simulink model "A8_Problem_1"  (R2023b)
settings: Solver=VariableStepAuto  StartTime=0.0  StopTime=t  FixedStep=dt  RelTol=1e-3
undefined symbols (not defined in the file): A1, A2, alpha, angle_threshold, beta, g, Gamma, K, k, l, lambda_0, lambda_1, m, q_0, q_dot_0, sat_limit, switch_time, theta_0, useEstimates, w1, w2
settings Model: Creator=eliasoa  LastModifiedBy=eliasoa

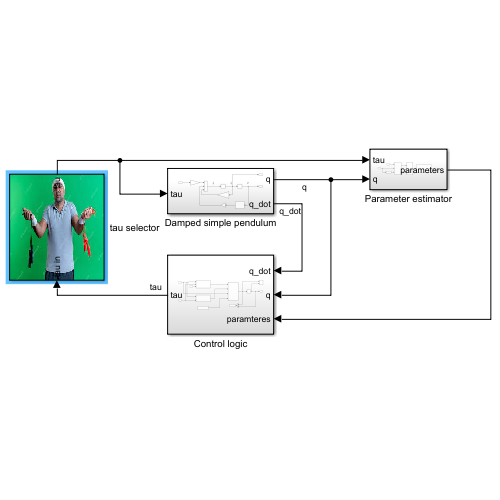
[thumbnail: Simulink's stored preview of the top-level diagram]
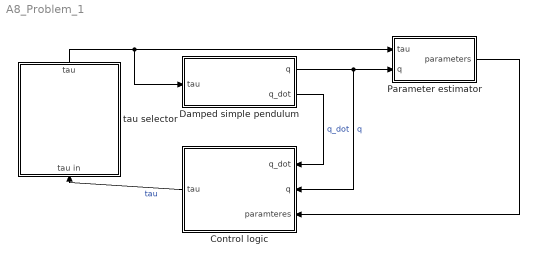
== system A8_Problem_1 ==
  Control logic : Subsystem
  Damped simple pendulum : Subsystem
  Parameter estimator : Subsystem
  "tau selector " : Subsystem
      mask Display: image('two tau.jpg');
  wires:
  Damped simple pendulum/1(q) -> Control logic/2(q), Parameter estimator/2(q)  "q"
  Damped simple pendulum/2(q_dot) -> Control logic/1(q_dot)  "q_dot"
  Parameter estimator/1(parameters) -> Control logic/3(paramteres)
  "tau selector "/1(tau) -> Damped simple pendulum/1(tau), Parameter estimator/1(tau)
  Control logic/1(tau) -> "tau selector "/1(tau in)  "tau"

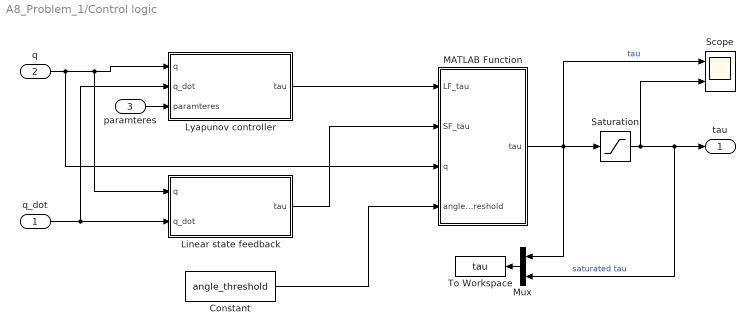
== system A8_Problem_1/Control logic ==
  q_dot : Inport
  q : Inport  Port=2
  paramteres : Inport  Port=3
  Constant : Constant  Value=angle_threshold
  Linear state feedback : Subsystem
  Lyapunov controller : Subsystem
  MATLAB Function : MATLAB Function  TreatAsAtomicUnit=on
  Mux : Mux  Inputs=2
  Saturation : Saturate  UpperLimit=sat_limit  LowerLimit=-sat_limit
  Scope : Scope  NumInputPorts=2
  To Workspace : ToWorkspace  VariableName=tau  SaveFormat=Timeseries  SampleTime=-1
  tau : Outport
  wires:
  q/1 -> Lyapunov controller/1(q), Linear state feedback/1(q), MATLAB Function/3(q)
  q_dot/1 -> Lyapunov controller/2(q_dot), Linear state feedback/2(q_dot)
  Linear state feedback/1(tau) -> MATLAB Function/2(SF_tau)
  Lyapunov controller/1(tau) -> MATLAB Function/1(LF_tau)
  MATLAB Function/1(tau) -> Saturation/1, Mux/1, Scope/1  "tau"
  Saturation/1 -> Scope/2, Mux/2, tau/1  "saturated tau"
  Mux/1 -> To Workspace/1
  Constant/1 -> MATLAB Function/4(angle_threshold)
  paramteres/1 -> Lyapunov controller/3(paramteres)

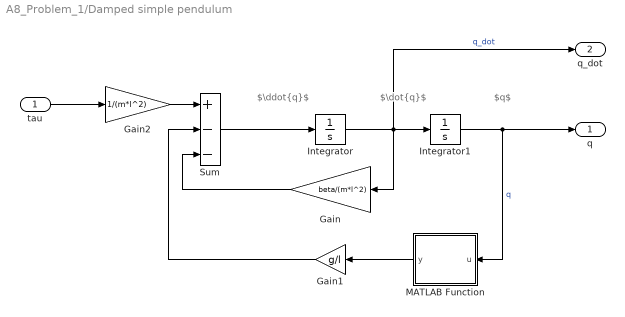
== system A8_Problem_1/Damped simple pendulum ==
  note: $\ddot{q}$
  note: $\dot{q}$
  note: $q$
  tau : Inport
  Gain : Gain  Gain=beta/(m*l^2)
  Gain1 : Gain  Gain=g/l
  Gain2 : Gain  Gain=1/(m*l^2)
  Integrator : Integrator  InitialCondition=q_dot_0
  Integrator1 : Integrator  InitialCondition=q_0
  MATLAB Function : MATLAB Function  TreatAsAtomicUnit=on
  Sum : Sum  Inputs=+--
  q : Outport
  q_dot : Outport  Port=2
  wires:
  tau/1 -> Gain2/1
  Sum/1 -> Integrator/1
  Gain2/1 -> Sum/1
  Gain/1 -> Sum/3
  MATLAB Function/1(y) -> Gain1/1
  Gain1/1 -> Sum/2
  Integrator/1 -> Integrator1/1, q_dot/1, Gain/1  "q_dot"
  Integrator1/1 -> q/1, MATLAB Function/1(u)  "q"

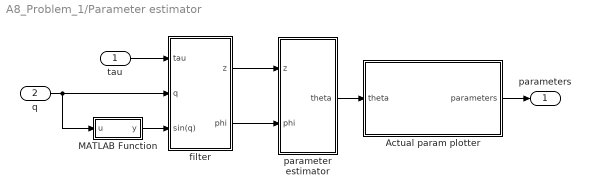
== system A8_Problem_1/Parameter estimator ==
  tau : Inport
  q : Inport  Port=2
  Actual param plotter : Subsystem
      mask Display: image('Kowalski.jpg');
  MATLAB Function : MATLAB Function  TreatAsAtomicUnit=on
  filter : Subsystem
  parameter estimator : Subsystem
  parameters : Outport
  wires:
  q/1 -> MATLAB Function/1(u), filter/2(q)
  tau/1 -> filter/1(tau)
  parameter estimator/1(theta) -> Actual param plotter/1(theta)
  filter/2(phi) -> parameter estimator/2(phi)
  Actual param plotter/1(parameters) -> parameters/1
  filter/1(z) -> parameter estimator/1(z)
  MATLAB Function/1(y) -> filter/3(sin(q))

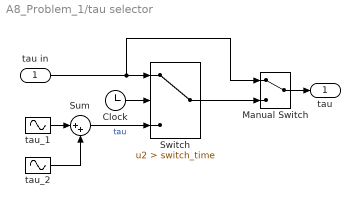
== system A8_Problem_1/tau selector  ==
  tau in : Inport
  Clock : Clock
  Manual Switch : ManualSwitch
  Sum : Sum  Inputs=|++
  Switch : Switch  Criteria=u2 > Threshold  Threshold=switch_time  SaturateOnIntegerOverflow=off  InputSameDT=off
  tau_1 : Sin  Amplitude=A1  Frequency=w1  SampleTime=0
  tau_2 : Sin  Amplitude=A2  Frequency=w2  SampleTime=0
  tau : Outport
  wires:
  tau in/1 -> Manual Switch/1, Switch/1
  tau_2/1 -> Sum/2
  tau_1/1 -> Sum/1
  Switch/1 -> Manual Switch/2
  Sum/1 -> Switch/3  "tau"
  Clock/1 -> Switch/2
  Manual Switch/1 -> tau/1

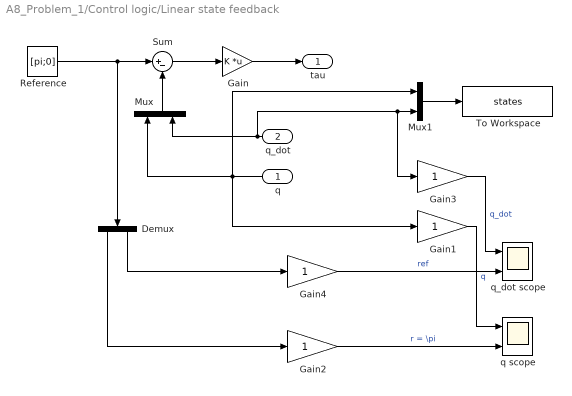
== system A8_Problem_1/Control logic/Linear state feedback ==
  q : Inport
  q_dot : Inport  Port=2
  Demux : Demux  Outputs=2
  Gain : Gain  Gain=K  Multiplication=Matrix(K*u)
  Gain{1..4} (4 alike) : Gain
  Mux : Mux  Inputs=2
  Mux1 : Mux  Inputs=2
  Reference : Constant  Value=[pi;0]
  Sum : Sum  Inputs=|+-
  To Workspace : ToWorkspace  VariableName=states  SaveFormat=Timeseries  SampleTime=-1
  q scope : Scope  NumInputPorts=2
  q_dot scope : Scope  NumInputPorts=2
  tau : Outport
  wires:
  Sum/1 -> Gain/1
  Mux/1 -> Sum/2
  Demux/2 -> Gain4/1
  q_dot/1 -> Gain3/1, Mux1/2, Mux/2
  q/1 -> Gain1/1, Mux/1, Mux1/1
  Demux/1 -> Gain2/1
  Reference/1 -> Sum/1, Demux/1
  Gain1/1 -> q scope/1  "q"
  Gain2/1 -> q scope/2  "r = \\pi"
  Gain/1 -> tau/1
  Mux1/1 -> To Workspace/1
  Gain4/1 -> q_dot scope/2  "ref"
  Gain3/1 -> q_dot scope/1  "q_dot"

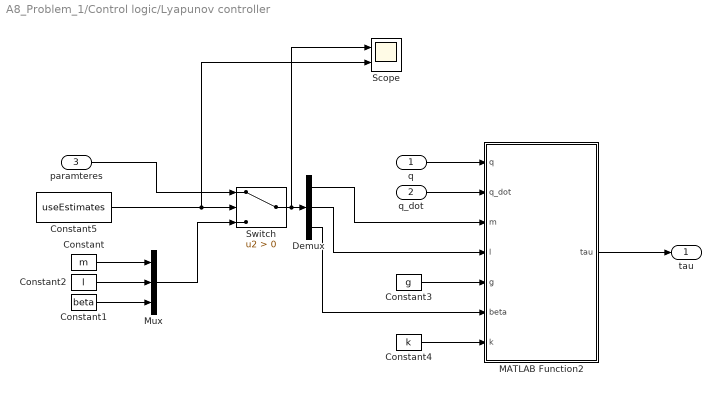
== system A8_Problem_1/Control logic/Lyapunov controller ==
  q : Inport
  q_dot : Inport  Port=2
  paramteres : Inport  Port=3
  Constant : Constant  Value=m
  Constant1 : Constant  Value=beta
  Constant2 : Constant  Value=l
  Constant3 : Constant  Value=g
  Constant4 : Constant  Value=k
  Constant5 : Constant  Value=useEstimates
  Demux : Demux  Outputs=3
  MATLAB Function2 : MATLAB Function  TreatAsAtomicUnit=on
  Mux : Mux  Inputs=3
  Scope : Scope  NumInputPorts=2
  Switch : Switch  Criteria=u2 > Threshold  SaturateOnIntegerOverflow=off  InputSameDT=off
  tau : Outport
  wires:
  MATLAB Function2/1(tau) -> tau/1
  Constant3/1 -> MATLAB Function2/5(g)
  q/1 -> MATLAB Function2/1(q)
  q_dot/1 -> MATLAB Function2/2(q_dot)
  Constant4/1 -> MATLAB Function2/7(k)
  paramteres/1 -> Switch/1
  Constant5/1 -> Scope/2, Switch/2
  Switch/1 -> Scope/1, Demux/1
  Mux/1 -> Switch/3
  Constant2/1 -> Mux/2
  Constant/1 -> Mux/1
  Constant1/1 -> Mux/3
  Demux/1 -> MATLAB Function2/3(m)
  Demux/2 -> MATLAB Function2/4(l)
  Demux/3 -> MATLAB Function2/6(beta)

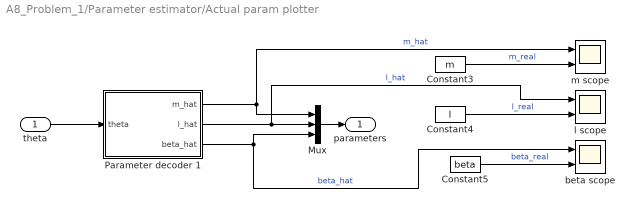
== system A8_Problem_1/Parameter estimator/Actual param plotter ==
  theta : Inport
  Constant3 : Constant  Value=m
  Constant4 : Constant  Value=l
  Constant5 : Constant  Value=beta
  Mux : Mux  Inputs=3
  Parameter decoder 1 : MATLAB Function  TreatAsAtomicUnit=on
  beta scope : Scope  NumInputPorts=2
  l scope : Scope  NumInputPorts=2
  m scope : Scope  NumInputPorts=2
  parameters : Outport
  wires:
  theta/1 -> Parameter decoder 1/1(theta)
  Parameter decoder 1/3(beta_hat) -> Mux/3, beta scope/1  "beta_hat"
  Parameter decoder 1/1(m_hat) -> Mux/1, m scope/1  "m_hat"
  Parameter decoder 1/2(l_hat) -> Mux/2, l scope/1  "l_hat"
  Constant5/1 -> beta scope/2  "beta_real"
  Constant3/1 -> m scope/2  "m_real"
  Constant4/1 -> l scope/2  "l_real"
  Mux/1 -> parameters/1

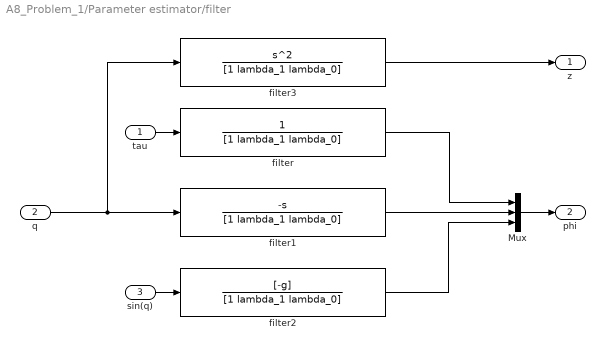
== system A8_Problem_1/Parameter estimator/filter ==
  tau : Inport
  q : Inport  Port=2
  sin(q) : Inport  Port=3
  Mux : Mux  Inputs=3
  filter : TransferFcn  Denominator=[1 lambda_1 lambda_0]
  filter1 : TransferFcn  Numerator=[-1 0]  Denominator=[1 lambda_1 lambda_0]
  filter2 : TransferFcn  Numerator=[-g]  Denominator=[1 lambda_1 lambda_0]
  filter3 : TransferFcn  Numerator=[1 0 0]  Denominator=[1 lambda_1 lambda_0]
  z : Outport
  phi : Outport  Port=2
  wires:
  filter1/1 -> Mux/2
  filter2/1 -> Mux/3
  filter/1 -> Mux/1
  sin(q)/1 -> filter2/1
  tau/1 -> filter/1
  q/1 -> filter3/1, filter1/1
  Mux/1 -> phi/1
  filter3/1 -> z/1

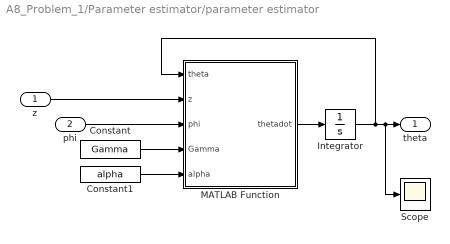
== system A8_Problem_1/Parameter estimator/parameter estimator ==
  z : Inport
  phi : Inport  Port=2
  Constant : Constant  Value=Gamma
  Constant1 : Constant  Value=alpha
  Integrator : Integrator  InitialCondition=theta_0
  MATLAB Function : MATLAB Function  TreatAsAtomicUnit=on
  Scope : Scope
  theta : Outport
  wires:
  Constant1/1 -> MATLAB Function/5(alpha)
  Integrator/1 -> Scope/1, theta/1, MATLAB Function/1(theta)
  phi/1 -> MATLAB Function/3(phi)
  MATLAB Function/1(thetadot) -> Integrator/1
  z/1 -> MATLAB Function/2(z)
  Constant/1 -> MATLAB Function/4(Gamma)

== matlab function A8_Problem_1/Parameter estimator/MATLAB Function ==
  data: u input; y output
function y = fcn(u)

y = sin(u);

== matlab function A8_Problem_1/Control logic/MATLAB Function ==
  data: LF_tau input; tau output; SF_tau input; q input; angle_threshold input
function tau = ControlSwitch(LF_tau, SF_tau,q,angle_threshold)

if q >= angle_threshold
    tau = SF_tau;
else
    tau = LF_tau;
end

== matlab function A8_Problem_1/Control logic/Lyapunov controller/MATLAB Function2 ==
  data: q input; tau output; q_dot input; m input; l input; g input; beta input; k input
function tau = tau(q,q_dot,m,l,g,beta,k)
E =1/2 * m * l^2 * q_dot^2 + m * g * l * ( 1 - cos(q) );
E_d = 2 * m * g * l;
TildeE = E-E_d;
tau = -k*TildeE*q_dot + beta*q_dot;

== matlab function A8_Problem_1/Damped simple pendulum/MATLAB Function ==
  data: u input; y output
function y = sin(u)

y = sin(u);

== matlab function A8_Problem_1/Parameter estimator/parameter estimator/MATLAB Function ==
  data: theta input; thetadot output; z input; phi input; Gamma input; alpha input
function thetadot = fcn(theta,z,phi,Gamma,alpha)
m2 = 1 + alpha*(phi'*phi);
epsilon = (z-theta'*phi)/m2;
thetadot = Gamma * epsilon * phi;

== matlab function A8_Problem_1/Parameter estimator/Actual param plotter/Parameter decoder 1 ==
  data: theta input; m_hat output; l_hat output; beta_hat output
function [m_hat,l_hat,beta_hat] = fcn(theta)
theta_1 = theta(1); %  1 / ml^2
theta_2 = theta(2); % β / ml^2
theta_3 = theta(3); % 1 / l

m_hat= theta_3^2/(theta_1);
l_hat = 1/theta_3;
beta_hat= theta_2/theta_1;
